simulink model "Pacemaker_1"  (R2020a)
settings: Solver=FixedStepAuto  StartTime=0.0  StopTime=10.0  FixedStep=1e-3  RelTol=1e-3  EnableMultiTasking=on
undefined symbols (not defined in the file or in its folder): D10, D11, D12, D13, D2, D3, D4, D5, D6, D7, D8, D9, PTA0, PTA1, PTA2, PTB23, PTB9, PTC2, PTC3, PTC4, PTD0, PTD1, PTD2, PTD3
libraries: frdmk64flib x15
settings Model: ExtModeTrigDuration=5  Creator=Udeep  LastModifiedBy=changhaibian
settings OptimizationCC: EnhancedBackFolding=on  PassReuseOutputArgsAs=Individual arguments  ZeroExternalMemoryAtStartup=off  ZeroInternalMemoryAtStartup=off  MaxStackSize=64  OptimizeBlockOrder=speed  DifferentSizesBufferReuse=on  OptimizationCustomize=off  EfficientTunableParamExpr=on
settings DebuggingCC: ParameterTunabilityLossMsg=error
settings HardwareCC: ProdBitPerPointer=32  ProdBitPerSizeT=32  ProdBitPerPtrDiffT=32  ProdLargestAtomicInteger=Long  ProdLargestAtomicFloat=Double  ProdWordSize=32  ProdHWDeviceType=ARM Compatible->ARM Cortex
settings SFSimCC: MATLABDynamicMemAlloc=off
settings RTWCC: SystemTargetFile=ert.tlc  HardwareBoard=NXP FRDM-K64F  TemplateMakefile=ert_default_tmf  Toolchain=GNU Tools for ARM Embedded Processors
settings CodeAppCC: ForceParamTrailComments=on  IgnoreCustomStorageClasses=off  OperatorAnnotations=on  SimulinkDataObjDesc=on  SFDataObjDesc=on  InsertBlockDesc=on

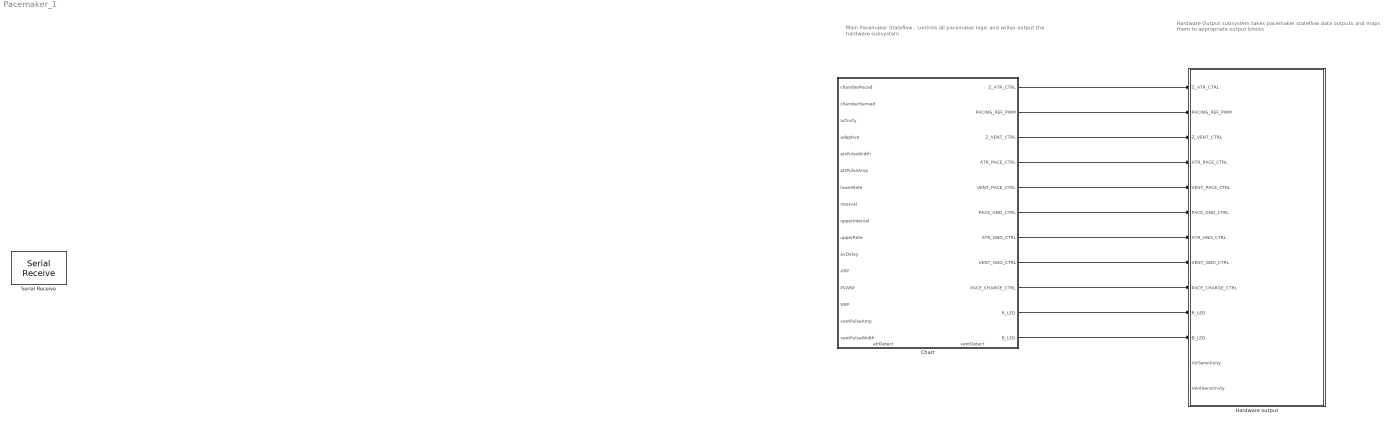
== system Pacemaker_1 ==
  note: Hardware Output subsystem takes pacemaker stateflow data outputs and maps them to appropriate output blocks
  note: Main Pacemaker Stateflow , controls all pacemaker logic and writes output the hardware subsystem
  Chart : Stateflow chart  TreatAsAtomicUnit=on
      settings: PortSchema="{\"entries\":[{\"content\":{\"sides\":[{\"content\":{\"connectorIds\":[\"In4\",\"In6\",\"In7\",\"In5\",\"In8\",\"In9\",\"In17\",\"In10\",\"In11\",\"In18\",\"In12\",\"In13\",\"In16\",\"In1\",\"In14\",\"In15\"]},\"type\":\"ConnectorPlacement.EquallySpacedRectSide\",\"uuid\":\"0f4bb13e-4f4f-48e2-b63c-32132ec29449\"},{\"content\":{\"connectorIds\":[\"Out1\",\"Out2\",\"Out3\",\"Out4\",\"Out5\",\"Out6\",\"Out7\",\"Out8\",\"Out9\",\"Out10\",\"Out11\"],\"side\":\"RIGHT\"},\"type\":\"ConnectorPlacement.EquallySpacedRectSide\",\"uuid\":\"66676ed7-b2a9-4718-87b6-7ef1563d11ef\"},{\"content\":{\"connectorIds\":[],\"side\":\"TOP\"},\"type\":\"ConnectorPlacement.EquallySpacedRectSide\",\"uuid\":\"f8ed3d2c-017d-4860-9941-e982831d4406\"},{\"content\":{\"connectorIds\":[\"In2\",\"In3\"],\"side\":\"BOTTOM\"},\"type\":\"ConnectorPlacement.EquallySpacedRectSide\",\"uuid\":\"e6b63469-3180-4838-a33b-c03ead75d417\"}]},\"type\":\"ConnectorPlacement.EquallySpacedConnector\",\"uuid\":\"d1db759d-e7ed-4d4b-bc59-5cab093840d4\"}],\"packageUris\":[\"http://schema.mathworks.com/mf0/Connector/19700101\"],\"version\":\"1.0\"}"
  Hardware output : Subsystem
  Serial Receive : frdmk64flib/Serial Receive  SCIModule=0  Baudrate=uint32(9600)  Parity=None  StopBits=1  HardwareFlowControl=None  ByteOrder=LittleEndian  DataType=uint8  DataLength=34  BlockingMode=off  OutputStatus=on  SampleTime=-1
  wires:
  Chart/9(PACE_CHARGE_CTRL) -> Hardware output/9(PACE_CHARGE_CTRL)
  Chart/1(Z_ATR_CTRL) -> Hardware output/1(Z_ATR_CTRL)
  Chart/5(VENT_PACE_CTRL) -> Hardware output/5(VENT_PACE_CTRL)
  Chart/3(Z_VENT_CTRL) -> Hardware output/3(Z_VENT_CTRL)
  Chart/4(ATR_PACE_CTRL) -> Hardware output/4(ATR_PACE_CTRL)
  Chart/10(R_LED) -> Hardware output/10(R_LED)
  Chart/7(ATR_GND_CTRL) -> Hardware output/7(ATR_GND_CTRL)
  Chart/6(PACE_GND_CTRL) -> Hardware output/6(PACE_GND_CTRL)
  Chart/11(B_LED) -> Hardware output/11(B_LED)
  Chart/8(VENT_GND_CTRL) -> Hardware output/8(VENT_GND_CTRL)
  Chart/2(PACING_REF_PWM) -> Hardware output/2(PACING_REF_PWM)

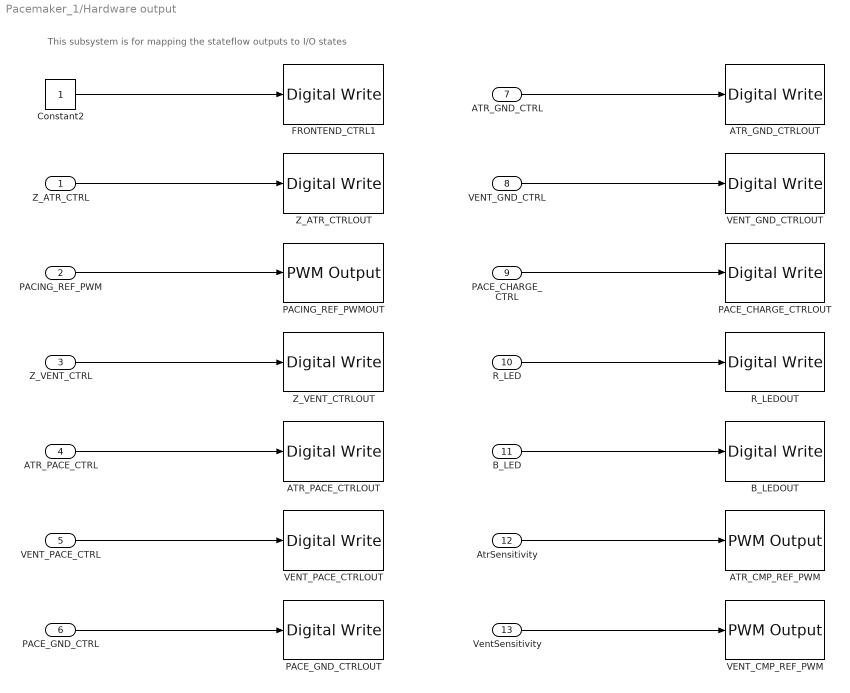
== system Pacemaker_1/Hardware output ==
  note: This subsystem is for mapping the stateflow outputs to I/O states
  Z_ATR_CTRL : Inport
  PACING_REF_PWM : Inport  Port=2
  Z_VENT_CTRL : Inport  Port=3
  ATR_PACE_CTRL : Inport  Port=4
  VENT_PACE_CTRL : Inport  Port=5
  PACE_GND_CTRL : Inport  Port=6
  ATR_GND_CTRL : Inport  Port=7
  VENT_GND_CTRL : Inport  Port=8
  PACE_CHARGE_CTRL : Inport  Port=9
  R_LED : Inport  Port=10
  B_LED : Inport  Port=11
  AtrSensitivity : Inport  Port=12
  VentSensitivity : Inport  Port=13
  ATR_CMP_REF_PWM : frdmk64flib/PWM Output  Whichpin=PTC2 (D6)  InitialFrequency=2000  InitialDutyCycle=0
  ATR_GND_CTRLOUT : frdmk64flib/Digital Write  Whichpin=PTD2 (D11)
  ATR_PACE_CTRLOUT : frdmk64flib/Digital Write  Whichpin=PTA0 (D8)
  B_LEDOUT : frdmk64flib/Digital Write  Whichpin=BLUE_LED
  Constant2 : Constant
  FRONTEND_CTRL1 : frdmk64flib/Digital Write  Whichpin=PTD1 (D13)
  PACE_CHARGE_CTRLOUT : frdmk64flib/Digital Write  Whichpin=PTB9 (D2)
  PACE_GND_CTRLOUT : frdmk64flib/Digital Write  Whichpin=PTD0 (D10)
  PACING_REF_PWMOUT : frdmk64flib/PWM Output  Whichpin=PTA2 (D5)  InitialFrequency=2000  InitialDutyCycle=0
  R_LEDOUT : frdmk64flib/Digital Write  Whichpin=RED_LED
  VENT_CMP_REF_PWM : frdmk64flib/PWM Output  Whichpin=PTA1 (D3)  InitialFrequency=2000  InitialDutyCycle=0
  VENT_GND_CTRLOUT : frdmk64flib/Digital Write  Whichpin=PTD3 (D12)
  VENT_PACE_CTRLOUT : frdmk64flib/Digital Write  Whichpin=PTC4 (D9)
  Z_ATR_CTRLOUT : frdmk64flib/Digital Write  Whichpin=PTB23 (D4)
  Z_VENT_CTRLOUT : frdmk64flib/Digital Write  Whichpin=PTC3 (D7)
  wires:
  Constant2/1 -> FRONTEND_CTRL1/1
  Z_ATR_CTRL/1 -> Z_ATR_CTRLOUT/1
  PACING_REF_PWM/1 -> PACING_REF_PWMOUT/1
  Z_VENT_CTRL/1 -> Z_VENT_CTRLOUT/1
  ATR_PACE_CTRL/1 -> ATR_PACE_CTRLOUT/1
  VENT_PACE_CTRL/1 -> VENT_PACE_CTRLOUT/1
  PACE_GND_CTRL/1 -> PACE_GND_CTRLOUT/1
  ATR_GND_CTRL/1 -> ATR_GND_CTRLOUT/1
  VENT_GND_CTRL/1 -> VENT_GND_CTRLOUT/1
  PACE_CHARGE_CTRL/1 -> PACE_CHARGE_CTRLOUT/1
  R_LED/1 -> R_LEDOUT/1
  B_LED/1 -> B_LEDOUT/1
  AtrSensitivity/1 -> ATR_CMP_REF_PWM/1
  VentSensitivity/1 -> VENT_CMP_REF_PWM/1

== stateflow chart Pacemaker_1/Chart ==
  note: Init
      | This state is meant for any boot-up operations that need to occur once before normal operation.Intial pin configurations and the capacitor is pre-charged here.
  state INIT
    Z_ATR_CTRL = false;
    Z_VENT_CTRL = false;
    % selecting correct initial pulse amplitude
    if chamberPaced == ChamberPaced.VENTRICLE_P
    pulseAmp = ventPulseAmp;
    else
    pulseAmp = atrPulseAmp;
    end
    PACING_REF_PWM = (pulseAmp/5);
    ATR_PACE_CTRL = false;
    VENT_PACE_CTRL = false;
    PACE_GND_CTRL = true;
    ATR_GND_CTRL = false;
    VENT_GND_CTRL = false;
    PACE_CHARGE_CTRL = true;
    R_LED = false; %testing pin
    B_LED = false; %testing pin
  state Sense
    note: Loops back for sensed case in inhibited
    state Default
    note: Default exists to constantly check if the mode is the same or is changed.
    note: For DXXX or XDXX or AXXX or XAXX modes
    note: For VXXX or XVXX modes
    note: Loops back for sensed case in inhibited
    state Ventricle
      state Default
        ActiveChamber = 2;
        %Update pace params to chamber
        pulseWidth = ventPulseWidth
        pulseAmp = ventPulseAmp
      note: Sets the active chamber, which directs where to pace
          | 1 = Atrium
          | 2 = Ventrical
      state Inhibited_VRP
        %Waits for VRP before sensing
      state None
        %Wait for a time then pace
      state Inhibited
        %checks if the heart paced
      state PaceSend
        %Sends to Pace
        send(paceStart)
      (default) -> Sense.Ventricle.Default
      Sense.Ventricle.Default -> (junction 147)
      (junction 147) -> Inhibited_VRP [order 1] : [activity == Activity.INHIBITED_A]
      (junction 147) -> Sense.Ventricle.None [order 2] : [activity == Activity.NONE_A]
      Inhibited_VRP -> Inhibited : after(VRP-pulseWidth,msec)
      Sense.Ventricle.None -> Sense.Ventricle.PaceSend [order 2] : after(interval-pulseWidth,msec)
      Sense.Ventricle.None -> Sense.Ventricle.PaceSend [order 1] : [after(avDelay,msec) && dualSense(chamberPaced,chamberSensed)]
      Inhibited -> Sense.Ventricle.PaceSend [order 1] : after(interval-VRP,msec)
    note: Fired from Pace after a pulse is sent and if ventricular sensing still needs to occur for XDXX and DXXX modes
    state Atrium
      state Default
        ActiveChamber = 1;
        %Update pace params to chamber
        pulseWidth = atrPulseWidth
        pulseAmp = atrPulseAmp
      note: Sets the active chamber, which directs where to pace
          | 1 = Atrium
          | 2 = Ventrical
      note: Junction detects the activity modes
      state Tiggered [commented out]
        %code for detecting Pwave
        %if found executes
        %send(V_PaceBypass)
        %meant for Dual modes
      state Inhibited_ARP
        %Waits for ARP before sensing
      state None
        %Wait then pace
      state InhibitedSense
        %checks if the heart paced
      state PaceSend
        %sends to pace
        send(paceStart)
      (default) -> Sense.Atrium.Default
      Sense.Atrium.Default -> (junction 135)
      (junction 135) -> Sense.Atrium.None [order 1] : [activity == Activity.NONE_A]
      (junction 135) -> Tiggered [commented out] : [activity == Activity.DUAL_A]
      (junction 135) -> Inhibited_ARP [order 2] : [activity == Activity.INHIBITED_A]
      Inhibited_ARP -> InhibitedSense : after(ARP,msec)
      Sense.Atrium.None -> Sense.Atrium.PaceSend [order 2] : [after(interval-pulseWidth,msec)]
      Sense.Atrium.None -> Sense.Atrium.PaceSend [order 1] : [after((interval-avDelay-atrPulseWidth-ventPulseWidth),msec) && dualSense(chamberPaced,chamberSensed)]
      InhibitedSense -> Sense.Atrium.PaceSend [order 1] : after(interval-ARP,msec)
    note: Senses the Atrium
    note: Senses the Ventricle
    note: Function to validate transistion between Default and Ventricle
    note: Function to validate transistion between Default and Atrium
    InhibitedSense -> Sense.Default [order 2] : [atrDetect == true]
    Inhibited -> Sense.Default [order 2] : [ventDetect == true]/{after(pulseWidth,msec)}
    (default) -> Sense.Default
    Sense.Default -> Ventricle [order 1] : [ventSense(chamberPaced,chamberSensed)==1]
    Sense.Default -> Atrium [order 2] : [atrSense(chamberPaced,chamberSensed)==1]
  note: SenseStateflow
      | Holds the logic for sensing heart activity and responding to it. The letter code is considered before branching deeper based on the chamber sensed
  note: Function used to determine if in dual mode operation
  note: Bypass used for DXXX modes
  state Pace
    state Charging
      %Discharging Blocking Capacitor C21
      PACE_GND_CTRL = true;
      VENT_PACE_CTRL = false;
      ATR_PACE_CTRL = false;
      if(ActiveChamber == 1)
      ATR_GND_CTRL = true;
      VENT_GND_CTRL = false;
      else
      ATR_GND_CTRL = false;
      VENT_GND_CTRL = true;
      end
      %Sets the Charging of C22
      PACING_REF_PWM = (pulseAmp/5); %pulseAmp
      PACE_CHARGE_CTRL = true;
      send(paceEnd)
    note: Determines chamber to be paced
    state paceAtr
      ATR_PACE_CTRL = true;
    state Discharging
      %Pacing the active chamber
      PACE_CHARGE_CTRL = false;
      PACE_GND_CTRL = true;
      ATR_GND_CTRL = false;
      VENT_GND_CTRL = false;
    state paceVent
      VENT_PACE_CTRL = true;
    note: Setup pins before pacing a chamber
    note: Creates a recharge pulse and charges up the charging
        | capacitor for the next pace
    (default) -> Discharging
    paceAtr -> Charging : after(pulseWidth,msec)
    Discharging -> paceAtr [order 1] : [ActiveChamber == 1]
    paceVent -> Charging : after(pulseWidth,msec)
    Discharging -> paceVent [order 2] : [ActiveChamber == 2]
  note: PaceStateflow
      | Triggered by an event from inside the sense stateflow to immediately discharge the pacing capacitor to the relevant chamber
      | Afterwards it will then trigger the charging state to manipulate the relevant IO to sink the blocking capacitor, and charge the pacing capacitor
      | As IO will be determined by the charging state before leaving this stateflow, the pacing capacitor is always effectively pre-charged
  (junction 278) -> Ventricle [order 1] : [dualSense(chamberPaced,chamberSensed) && ActiveChamber == 1]
  (default) -> INIT
  INIT -> Sense
  Sense -> Pace : paceStart
  (junction 278) -> Sense [order 2]
  Pace -> (junction 278) : paceEnd
  data: a function_input; b function_input; v function_output; v function_output; a function_input; b function_input; a function_input; b function_input; v function_output; Z_ATR_CTRL output; VRP input; atrDetect input boolean; ventDetect input boolean; chamberPaced input; adaptive input; chamberSensed input; activity input; atrPulseWidth input; atrPulseAmp input; interval input; upperInterval input; avDelay input; ARP input; ventPulseAmp input; ventPulseWidth input; PVARP input; lowerRate input; upperRate input; PACING_REF_PWM output; Z_VENT_CTRL output; ATR_PACE_CTRL output; VENT_PACE_CTRL output; PACE_GND_CTRL output; ATR_GND_CTRL output; VENT_GND_CTRL output; PACE_CHARGE_CTRL output; R_LED output boolean; B_LED output boolean; ActiveChamber local; iniTime local; pulseWidth local; pulseAmp local
  events: paceStart local FUNCTION_CALL_EVENT; paceEnd local FUNCTION_CALL_EVENT; dischargePace local RISING_EDGE_EVENT; chargePace local RISING_EDGE_EVENT; V_PaceBypass local FUNCTION_CALL_EVENT; AtrSense local FUNCTION_CALL_EVENT; VentSense local FUNCTION_CALL_EVENT; V_Loop local FUNCTION_CALL_EVENT; A_Loop local FUNCTION_CALL_EVENT; Vent_Bypass local FUNCTION_CALL_EVENT
  function v = ventSense(a,b):
    | function  v = ventSense(a,b)
    |     if (a == ChamberPaced.VENTRICLE_P)
    |         v = 1;
    |     elseif (b == ChamberSensed.VENTRICLE_S)
    |         v = 1;
    |     else
    |         v = 0;
    |     end
    | end
  function v = atrSense(a,b):
    | function v = atrSense(a,b)
    |     if (a == ChamberPaced.ATRIUM_P)
    |         v = 1;
    |     elseif (a == ChamberPaced.DUAL_P)
    |         v = 1;
    |     elseif (b == ChamberSensed.ATRIUM_S)
    |         v = 1;
    |     elseif (b == ChamberSensed.DUAL_S)
    |         v = 1;
    |     else
    |         v = 0;
    |     end
    | end
  function v = dualSense(a,b):
    | function v = dualSense(a,b)
    |     if (a == ChamberPaced.DUAL_P)
    |         v = 1;
    |     elseif (b == ChamberSensed.DUAL_S)
    |         v = 1;
    |     else
    |         v = 0;
    |     end
    | end
